simulink model "class_7_simulink"  (R2023b)
settings: Solver=VariableStepAuto  StartTime=0.0  StopTime=10.0  RelTol=1e-3
values from neighbouring files (symbols this model uses):
  denp = [3 1]    [class_7.m]
  h = 6.5    [class_7.m]
  nump = 2    [class_7.m]
libraries: cstblocks x6
settings Model: Creator=klysm  LastModifiedBy=klysm

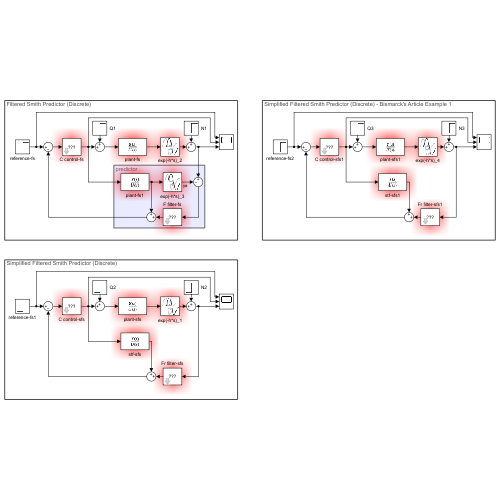
[thumbnail: Simulink's stored preview of the top-level diagram]
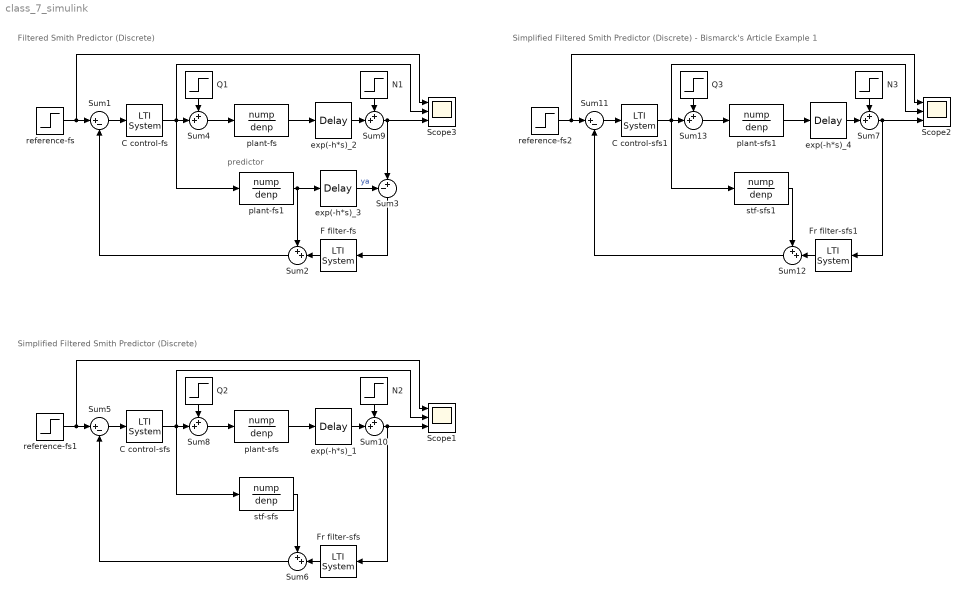
== system class_7_simulink ==
  note: Filtered Smith Predictor (Discrete)
  note: predictor
  note: Simplified Filtered Smith Predictor (Discrete)
  note: Simplified Filtered Smith Predictor (Discrete) - Bismarck's Article Example 1
  C control-fs : cstblocks/LTI System  sys=C  IC=[]  PadeOrder=0
  C control-sfs : cstblocks/LTI System  sys=C  IC=[]  PadeOrder=0
  C control-sfs1 : cstblocks/LTI System  sys=C  IC=[]  PadeOrder=0
  F filter-fs : cstblocks/LTI System  sys=C  IC=[]  PadeOrder=0
  Fr filter-sfs : cstblocks/LTI System  sys=C  IC=[]  PadeOrder=0
  Fr filter-sfs1 : cstblocks/LTI System  sys=C  IC=[]  PadeOrder=0
  N1 : Step  Time=25  After=0.2  SampleTime=0
  N2 : Step  Time=25  After=0.2  SampleTime=0
  N3 : Step  Time=25  After=0.2  SampleTime=0
  Q1 : Step  Time=12  SampleTime=0
  Q2 : Step  Time=12  SampleTime=0
  Q3 : Step  Time=12  SampleTime=0
  Scope1 : Scope  NumInputPorts=3
  Scope2 : Scope  NumInputPorts=3
  Scope3 : Scope  NumInputPorts=3
  Sum1 : Sum  Inputs=|+-
  Sum{2,4,6..10,12..13} (9 alike) : Sum  Inputs=++|
  Sum11 : Sum  Inputs=|+-
  Sum3 : Sum  Inputs=-+|
  Sum5 : Sum  Inputs=|+-
  exp(-h*s)_{1..4} (4 alike) : TransportDelay  DelayTime=h
  plant-fs : TransferFcn  Numerator=nump  Denominator=denp
  plant-fs1 : TransferFcn  Numerator=nump  Denominator=denp
  plant-sfs : TransferFcn  Numerator=nump  Denominator=denp
  plant-sfs1 : TransferFcn  Numerator=nump  Denominator=denp
  reference-fs : Step  SampleTime=0
  reference-fs1 : Step  SampleTime=0
  reference-fs2 : Step  SampleTime=0
  stf-sfs : TransferFcn  Numerator=nump  Denominator=denp
  stf-sfs1 : TransferFcn  Numerator=nump  Denominator=denp
  wires:
  Sum3/1 -> F filter-fs/1
  reference-fs/1 -> Scope3/1, Sum1/1
  plant-fs1/1 -> exp(-h*s)_3/1, Sum2/1
  plant-fs/1 -> exp(-h*s)_2/1
  Sum2/1 -> Sum1/2
  exp(-h*s)_3/1 -> Sum3/1  "ya"
  Sum4/1 -> plant-fs/1
  Sum1/1 -> C control-fs/1
  Q1/1 -> Sum4/1
  F filter-fs/1 -> Sum2/2
  C control-fs/1 -> Scope3/2, Sum4/2, plant-fs1/1
  N1/1 -> Sum9/1
  Sum9/1 -> Sum3/2, Scope3/3
  exp(-h*s)_2/1 -> Sum9/2
  exp(-h*s)_1/1 -> Sum10/2
  Sum10/1 -> Fr filter-sfs/1, Scope1/3
  C control-sfs/1 -> Scope1/2, Sum8/2, stf-sfs/1
  Q2/1 -> Sum8/1
  N2/1 -> Sum10/1
  Fr filter-sfs/1 -> Sum6/2
  Sum5/1 -> C control-sfs/1
  Sum6/1 -> Sum5/2
  plant-sfs/1 -> exp(-h*s)_1/1
  reference-fs1/1 -> Scope1/1, Sum5/1
  Sum8/1 -> plant-sfs/1
  stf-sfs/1 -> Sum6/1
  stf-sfs1/1 -> Sum12/1
  reference-fs2/1 -> Scope2/1, Sum11/1
  Sum13/1 -> plant-sfs1/1
  Sum12/1 -> Sum11/2
  N3/1 -> Sum7/1
  C control-sfs1/1 -> Scope2/2, Sum13/2, stf-sfs1/1
  Fr filter-sfs1/1 -> Sum12/2
  Q3/1 -> Sum13/1
  plant-sfs1/1 -> exp(-h*s)_4/1
  Sum11/1 -> C control-sfs1/1
  exp(-h*s)_4/1 -> Sum7/2
  Sum7/1 -> Fr filter-sfs1/1, Scope2/3
